simulink model "Robot4_SDT"  (R2025b)
settings: Solver=VariableStepAuto  StartTime=0.0  StopTime=10.0  RelTol=1e-3
values from neighbouring files (symbols this model uses):
  C_tile_force = 2*5*sqrt(K_tile_force*2.598*0.2*100)    [Satellite_Data.m]    (also in main.m)
  C_tile_torque = 2*1*sqrt(K_tile_torque*0.541266*100)*0.7    [Satellite_Data.m]    (also in main.m)
  CoM_variation_x = ureal('CoMx',0,"PlusMinus",[-10e-3 10e-3])    [Satellite_Data.m]
  CoM_variation_y = ureal('CoMy',0,"PlusMinus",[-10e-3 10e-3])    [Satellite_Data.m]
  CoM_variation_z = ureal('CoMz',0,"PlusMinus",[-20e-3 20e-3])    [Satellite_Data.m]
  Container_x = 1.5    [Satellite_Data.m]
  Container_z = sqrt(3)+0.5    [Satellite_Data.m]
  J_B_B = [J_B_Bxx J_B_Bxy J_B_Bxz;         J_B_Bxy J_B_Byy J_B_Byz;         J_B_Bxz J_B_Byz J_B_Bzz]    [Satellite_Data.m]
  J_C_C = [J_C_Cxx J_C_Cxy J_C_Cxz;         J_C_Cxy J_C_Cyy J_C_Cyz;         J_C_Cxz J_C_Cyz J_C_Czz]    [Satellite_Data.m]
  J_P_P = [J_P_Pxx J_P_Pxy J_P_Pxz;         J_P_Pxy J_P_Pyy J_P_Pyz;         J_P_Pxz J_P_Pyz J_P_Pzz]    [Satellite_Data.m]
  J_T_T = [J_T_Txx J_T_Txy J_T_Txz;          J_T_Txy J_T_Tyy J_T_Tyz;          J_T_Txz J_T_Tyz J_T_Tzz]    [Satellite_Data.m]
  K_tile_force = 2000/0.015    (= 133333.333333)    [Satellite_Data.m]    (also in main.m)
  K_tile_torque = 250/deg2rad(10)    [Satellite_Data.m]    (also in main.m)
  m_B = ureal('m_B',1000,'percent',10)    [Satellite_Data.m]
  m_C = ureal('m_C',500,'percent',10)    [Satellite_Data.m]
  m_P = ureal('m_P',50,'percent',2)    [Satellite_Data.m]
  m_T = ureal('m_T', m_nominal, 'percent', 2)    [Satellite_Data.m]
  robot = struct()    [Robotic_Arm_traj.m]    (also in Robotic_Arm_traj_no_energy.m; Satellite_Data.m; redundant_7dof_feasible_trajectory.m)
  Tile_z = 0.05    [Satellite_Data.m]
  unc_freq_boom = 10    [Satellite_Data.m]
undefined symbols (not defined in the file or in its folder): boom, InvDyn, InvDynAug, KIN, ureal, uss
libraries: SDTlibV1 x73, RCTblocks x39
(part 4 of 5)

== system Robot4_SDT/Tiles/Tile6/Variant Subsystem/Depose ==
  m_A : Inport
  m_C : Inport  Port=2
  m_T1 : Inport  Port=3
  m_T2 : Inport  Port=4
  m_EE : Inport  Port=5
  Constant : Constant
  Demux1 : Demux  Outputs=3
  Demux2 : Demux  Outputs=2
  Demux3 : Demux  Outputs=3
  Demux4 : Demux  Outputs=2
  Force : Subsystem
  Gain1 : Gain  Gain=-1
  Ground2 : Ground
  Integrator : Integrator
  Integrator1 : Integrator
  Mux : Mux
  Product : Product
  Product1 : Product
  Sum : Sum  Inputs=+-
  Sum1 : Sum  Inputs=|+-
  Terminator{,1..4} (5 alike) : Terminator
  Torque : Subsystem
  Zero : Constant  Value=zeros(6,1)  OutDataTypeStr=Inherit: Inherit via back propagation
  Zero1 : Constant  Value=zeros(6,1)  OutDataTypeStr=Inherit: Inherit via back propagation
  Zero2 : Constant  Value=zeros(6,1)  OutDataTypeStr=Inherit: Inherit via back propagation
  massless connection body : Subsystem  mask(Massless multi_port [6+18(n-1)]x[6(n-1)+18]){n=2, numinv=1, OP1=[0;0;0], OP2=[1.5 +sqrt(3)/2 0], OP3=[ureal('P3_y',1,'percent',10);0;0], OP4=[0;0;0], OP5=[0;0;0], OP6=[0;0;0], OP7=[0;0;0]}
      mask prompts: n "Number of ports"; numinv "Port (point) Pj: j="; OP1 "OP1 (3x1 vector, m)"; OP2 "OP2 (3x1 vector, m)"; OP3 "OP3 (3x1 vector, m)"; OP4 "OP4 (3x1 vector, m)"; OP5 "OP5 (3x1 vector,m)"; OP6 "OP6 (3x1 vector,m)"; OP7 "OP7 (3x1 vector,m)"
      mask help:
      | Massless body to transport wrenches and acceleration twists:
      | [6+18(n-1)]x[6(n-1)+18] gain from:
      |  * the motion vector at one point Pj; i.e. the parent port,
      |  * the wrenches applied to this massless body at the n-1 points Pi (i=1,..n, except j); i.e. the child ports
      | to:
      |  * the wrench applied at point Pj by this massless body,
      |  * the motion vectors at the other n-1  points Pi (i=1,..n, except j).
      |
      | 0: the reference point
      | Pi (i=1:n): the n given connection points or ports (1<n<8).
      |
      | All parameters are expressed in the body frame.
      | Each parameter can be an uncertain parameter declared with "ureal"
      mask init:
      | MasslessConnectionBodyAug
      mask Help: web('DocMassLessBody.html','-browser','-browser')
      mask TypeOptions n: 2 | 3 | 4 | 5 | 6 | 7
      mask TypeOptions numinv: 1 | 2 | 3 | 4 | 5 | 6 | 7
      mask DialogControl ParameterGroupVar Prompt: Main parameters
      mask DialogControl port1 Prompt: Port #1
      mask DialogControl port2 Prompt: #2
      mask DialogControl port3 Prompt: #3
      mask DialogControl port4 Prompt: #4
      mask DialogControl port5 Prompt: #5
      mask DialogControl port6 Prompt: #6
      mask DialogControl port7 Prompt: #7
      mask Display:
      | disp('Massless\n connection body\n [6+18(n-1)]x[6(n-1)+18]')
      | for ii=1:n+1
      |     if numinv==ii,
      |         port_label('output',ii,['Wbody/.,P',num2str(ii)])
      |         port_label('input', ii,['m_P',num2str(ii)])
      |     else
      |         port_label('input', ii,['W./body,P',num2str(ii)])
      |         port_label('output',ii,['m_P',num2str(ii)])
      |     end
      | end
  W_A : Outport
  W_C : Outport  Port=2
  W_T1 : Outport  Port=3
  W_T2 : Outport  Port=4
  W_EE : Outport  Port=5
  wires:
  Force/1(Mating) -> Product1/2
  Constant/1 -> Product/2, Product1/1
  Demux3/3 -> [Fz]
  Demux3/1 -> [Fx]
  Demux3/2 -> [Fy]
  Product/1 -> [T]
  Torque/1(Mating) -> Product/1
  Product1/1 -> Demux3/1
  Demux4/2 -> Torque/1(EA)
  Demux4/1 -> Force/1(pos)
  [T] -> Mux/4
  Demux1/3 -> Terminator3/1
  Integrator1/1 -> Demux4/1
  [Fy] -> Mux/2
  Demux1/1 -> Integrator/1
  Gain1/1 -> Demux1/1
  massless connection body/2(out2) -> Sum/1
  [Fz] -> Mux/3
  Sum1/1 -> massless connection body/2(in2)
  Mux/1 -> Sum1/2, W_T1/1
  Demux1/2 -> Terminator2/1
  Demux2/2 -> Torque/2(Omega)
  [Fx] -> Mux/1
  Integrator/1 -> Demux2/1, Integrator1/1
  Ground2/1 -> Sum1/1
  Demux2/1 -> Force/2(vel)
  Sum/1 -> Gain1/1
  m_T1/1 -> Sum/2
  m_A/1 -> massless connection body/1(in1)
  massless connection body/1(out1) -> W_A/1
  m_T2/1 -> Terminator1/1
  m_EE/1 -> Terminator/1
  m_C/1 -> Terminator4/1
  Zero/1 -> W_EE/1
  Zero1/1 -> W_T2/1
  Zero2/1 -> W_C/1

== system Robot4_SDT/Tiles/Tile6/Variant Subsystem/Grab ==
  m_EE : Inport
  m_C : Inport  Port=2
  m_T2 : Inport  Port=3
  m_A : Inport  Port=4
  m_T1 : Inport  Port=5
  Demux1 : Demux  Outputs=3
  Demux2 : Demux  Outputs=2
  Demux3 : Demux  Outputs=3
  Demux4 : Demux  Outputs=2
  Force : Subsystem
  Gain1 : Gain  Gain=-1
  Ground2 : Ground
  Integrator : Integrator
  Integrator1 : Integrator
  Mux : Mux
  Sum : Sum  Inputs=+-
  Sum1 : Sum  Inputs=|+-
  Terminator{,1..4} (5 alike) : Terminator
  Torque : Subsystem
  Zero : Constant  Value=zeros(6,1)  OutDataTypeStr=Inherit: Inherit via back propagation
  Zero1 : Constant  Value=zeros(6,1)  OutDataTypeStr=Inherit: Inherit via back propagation
  Zero2 : Constant  Value=zeros(6,1)  OutDataTypeStr=Inherit: Inherit via back propagation
  massless connection body : Subsystem  mask(Massless multi_port [6+18(n-1)]x[6(n-1)+18]){n=2, numinv=1, OP1=[0;0;0], OP2=[0;0;0], OP3=[ureal('P3_y',1,'percent',10);0;0], OP4=[0;0;0], OP5=[0;0;0], OP6=[0;0;0], OP7=[0;0;0]}
      mask prompts: n "Number of ports"; numinv "Port (point) Pj: j="; OP1 "OP1 (3x1 vector, m)"; OP2 "OP2 (3x1 vector, m)"; OP3 "OP3 (3x1 vector, m)"; OP4 "OP4 (3x1 vector, m)"; OP5 "OP5 (3x1 vector,m)"; OP6 "OP6 (3x1 vector,m)"; OP7 "OP7 (3x1 vector,m)"
      mask help:
      | Massless body to transport wrenches and acceleration twists:
      | [6+18(n-1)]x[6(n-1)+18] gain from:
      |  * the motion vector at one point Pj; i.e. the parent port,
      |  * the wrenches applied to this massless body at the n-1 points Pi (i=1,..n, except j); i.e. the child ports
      | to:
      |  * the wrench applied at point Pj by this massless body,
      |  * the motion vectors at the other n-1  points Pi (i=1,..n, except j).
      |
      | 0: the reference point
      | Pi (i=1:n): the n given connection points or ports (1<n<8).
      |
      | All parameters are expressed in the body frame.
      | Each parameter can be an uncertain parameter declared with "ureal"
      mask init:
      | MasslessConnectionBodyAug
      mask Help: web('DocMassLessBody.html','-browser','-browser')
      mask TypeOptions n: 2 | 3 | 4 | 5 | 6 | 7
      mask TypeOptions numinv: 1 | 2 | 3 | 4 | 5 | 6 | 7
      mask DialogControl ParameterGroupVar Prompt: Main parameters
      mask DialogControl port1 Prompt: Port #1
      mask DialogControl port2 Prompt: #2
      mask DialogControl port3 Prompt: #3
      mask DialogControl port4 Prompt: #4
      mask DialogControl port5 Prompt: #5
      mask DialogControl port6 Prompt: #6
      mask DialogControl port7 Prompt: #7
      mask Display:
      | disp('Massless\n connection body\n [6+18(n-1)]x[6(n-1)+18]')
      | for ii=1:n+1
      |     if numinv==ii,
      |         port_label('output',ii,['Wbody/.,P',num2str(ii)])
      |         port_label('input', ii,['m_P',num2str(ii)])
      |     else
      |         port_label('input', ii,['W./body,P',num2str(ii)])
      |         port_label('output',ii,['m_P',num2str(ii)])
      |     end
      | end
  W_EE : Outport
  W_C : Outport  Port=2
  W_T2 : Outport  Port=3
  W_A : Outport  Port=4
  W_T1 : Outport  Port=5
  wires:
  Torque/1(Mating) -> [T]
  massless connection body/1(out1) -> W_EE/1
  m_EE/1 -> massless connection body/1(in1)
  m_T2/1 -> Sum/2
  Sum/1 -> Gain1/1
  Demux2/1 -> Force/2(vel)
  Ground2/1 -> Sum1/1
  Integrator/1 -> Integrator1/1, Demux2/1
  [Fx] -> Mux/1
  Demux2/2 -> Torque/2(Omega)
  Demux1/2 -> Terminator2/1
  Mux/1 -> W_T2/1, Sum1/2
  Sum1/1 -> massless connection body/2(in2)
  [Fz] -> Mux/3
  massless connection body/2(out2) -> Sum/1
  Gain1/1 -> Demux1/1
  Demux1/1 -> Integrator/1
  [Fy] -> Mux/2
  Integrator1/1 -> Demux4/1
  Demux1/3 -> Terminator3/1
  [T] -> Mux/4
  Demux4/1 -> Force/1(pos)
  Demux4/2 -> Torque/1(EA)
  Force/1(Mating) -> Demux3/1
  Demux3/2 -> [Fy]
  Demux3/1 -> [Fx]
  Demux3/3 -> [Fz]
  m_A/1 -> Terminator1/1
  m_C/1 -> Terminator/1
  m_T1/1 -> Terminator4/1
  Zero/1 -> W_C/1
  Zero1/1 -> W_A/1
  Zero2/1 -> W_T1/1

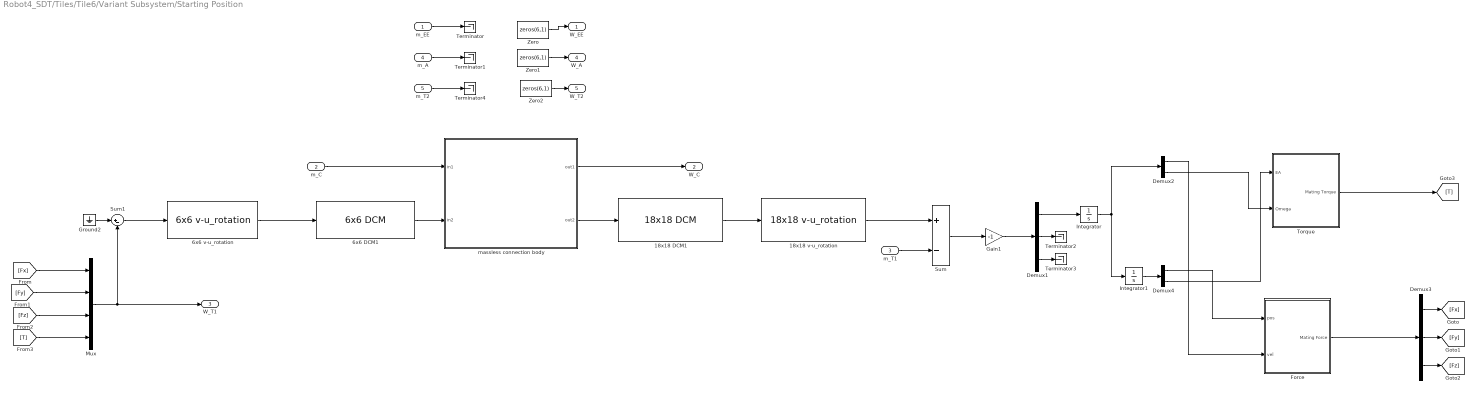
== system Robot4_SDT/Tiles/Tile6/Variant Subsystem/Starting Position ==
  m_EE : Inport
  m_C : Inport  Port=2
  m_T1 : Inport  Port=3
  m_A : Inport  Port=4
  m_T2 : Inport  Port=5
  18x18 DCM1 : SDTlibV1/3//6//18 DCM/18x18 DCM  rot=[0 0 1;0 1 0;-1 0 0]  transp=on
      settings: SourceProductName=SDTlib
  18x18 v-u_rotation : SDTlibV1/3//6//18 DCM/18x18 v-u_rotation  ra=[0;0;1]  theta=pi/2  transp=on
      settings: SourceProductName=SDTlib
  6x6 DCM1 : SDTlibV1/3//6//18 DCM/6x6 DCM  rot=[0 0 1;0 1 0;-1 0 0]  transp=off
      settings: SourceProductName=SDTlib
  6x6 v-u_rotation : SDTlibV1/3//6//18 DCM/6x6 v-u_rotation  ra=[0;0;1]  theta=pi/2  transp=off
      settings: SourceProductName=SDTlib
  Demux1 : Demux  Outputs=3
  Demux2 : Demux  Outputs=2
  Demux3 : Demux  Outputs=3
  Demux4 : Demux  Outputs=2
  Force : Subsystem
  Gain1 : Gain  Gain=-1
  Ground2 : Ground
  Integrator : Integrator
  Integrator1 : Integrator
  Mux : Mux
  Sum : Sum  Inputs=+-
  Sum1 : Sum  Inputs=|+-
  Terminator{,1..4} (5 alike) : Terminator
  Torque : Subsystem
  Zero : Constant  Value=zeros(6,1)  OutDataTypeStr=Inherit: Inherit via back propagation
  Zero1 : Constant  Value=zeros(6,1)  OutDataTypeStr=Inherit: Inherit via back propagation
  Zero2 : Constant  Value=zeros(6,1)  OutDataTypeStr=Inherit: Inherit via back propagation
  massless connection body : Subsystem  mask(Massless multi_port [6+18(n-1)]x[6(n-1)+18]){n=2, numinv=1, OP1=[0;0;0], OP2=[-1.2;0;0], OP3=[ureal('P3_y',1,'percent',10);0;0], OP4=[0;0;0], OP5=[0;0;0], OP6=[0;0;0], OP7=[0;0;0]}
      mask prompts: n "Number of ports"; numinv "Port (point) Pj: j="; OP1 "OP1 (3x1 vector, m)"; OP2 "OP2 (3x1 vector, m)"; OP3 "OP3 (3x1 vector, m)"; OP4 "OP4 (3x1 vector, m)"; OP5 "OP5 (3x1 vector,m)"; OP6 "OP6 (3x1 vector,m)"; OP7 "OP7 (3x1 vector,m)"
      mask help:
      | Massless body to transport wrenches and acceleration twists:
      | [6+18(n-1)]x[6(n-1)+18] gain from:
      |  * the motion vector at one point Pj; i.e. the parent port,
      |  * the wrenches applied to this massless body at the n-1 points Pi (i=1,..n, except j); i.e. the child ports
      | to:
      |  * the wrench applied at point Pj by this massless body,
      |  * the motion vectors at the other n-1  points Pi (i=1,..n, except j).
      |
      | 0: the reference point
      | Pi (i=1:n): the n given connection points or ports (1<n<8).
      |
      | All parameters are expressed in the body frame.
      | Each parameter can be an uncertain parameter declared with "ureal"
      mask init:
      | MasslessConnectionBodyAug
      mask Help: web('DocMassLessBody.html','-browser','-browser')
      mask TypeOptions n: 2 | 3 | 4 | 5 | 6 | 7
      mask TypeOptions numinv: 1 | 2 | 3 | 4 | 5 | 6 | 7
      mask DialogControl ParameterGroupVar Prompt: Main parameters
      mask DialogControl port1 Prompt: Port #1
      mask DialogControl port2 Prompt: #2
      mask DialogControl port3 Prompt: #3
      mask DialogControl port4 Prompt: #4
      mask DialogControl port5 Prompt: #5
      mask DialogControl port6 Prompt: #6
      mask DialogControl port7 Prompt: #7
      mask Display:
      | disp('Massless\n connection body\n [6+18(n-1)]x[6(n-1)+18]')
      | for ii=1:n+1
      |     if numinv==ii,
      |         port_label('output',ii,['Wbody/.,P',num2str(ii)])
      |         port_label('input', ii,['m_P',num2str(ii)])
      |     else
      |         port_label('input', ii,['W./body,P',num2str(ii)])
      |         port_label('output',ii,['m_P',num2str(ii)])
      |     end
      | end
  W_EE : Outport
  W_C : Outport  Port=2
  W_T1 : Outport  Port=3
  W_A : Outport  Port=4
  W_T2 : Outport  Port=5
  wires:
  Demux3/3 -> [Fz]
  Demux3/1 -> [Fx]
  Demux3/2 -> [Fy]
  Torque/1(Mating Torque) -> [T]
  Force/1(Mating Force) -> Demux3/1
  massless connection body/1(out1) -> W_C/1
  m_C/1 -> massless connection body/1(in1)
  m_T1/1 -> Sum/2
  Sum/1 -> Gain1/1
  Demux2/1 -> Force/2(vel)
  Ground2/1 -> Sum1/1
  Integrator/1 -> Integrator1/1, Demux2/1
  [Fx] -> Mux/1
  Demux2/2 -> Torque/2(Omega)
  Demux1/2 -> Terminator2/1
  Mux/1 -> Sum1/2, W_T1/1
  6x6 DCM1/1 -> massless connection body/2(in2)
  18x18 DCM1/1 -> 18x18 v-u_rotation/1
  Sum1/1 -> 6x6 v-u_rotation/1
  [Fz] -> Mux/3
  18x18 v-u_rotation/1 -> Sum/1
  Gain1/1 -> Demux1/1
  Demux1/1 -> Integrator/1
  6x6 v-u_rotation/1 -> 6x6 DCM1/1
  [Fy] -> Mux/2
  massless connection body/2(out2) -> 18x18 DCM1/1
  Integrator1/1 -> Demux4/1
  Demux1/3 -> Terminator3/1
  [T] -> Mux/4
  Demux4/1 -> Force/1(pos)
  Demux4/2 -> Torque/1(EA)
  m_A/1 -> Terminator1/1
  m_EE/1 -> Terminator/1
  m_T2/1 -> Terminator4/1
  Zero/1 -> W_EE/1
  Zero1/1 -> W_A/1
  Zero2/1 -> W_T2/1

== system Robot4_SDT/Tiles/Tile7/Variant Subsystem/Depose ==
  m_A : Inport
  m_C : Inport  Port=2
  m_T1 : Inport  Port=3
  m_T2 : Inport  Port=4
  m_EE : Inport  Port=5
  Constant : Constant
  Demux1 : Demux  Outputs=3
  Demux2 : Demux  Outputs=2
  Demux3 : Demux  Outputs=3
  Demux4 : Demux  Outputs=2
  Force : Subsystem
  Gain1 : Gain  Gain=-1
  Ground2 : Ground
  Integrator : Integrator
  Integrator1 : Integrator
  Mux : Mux
  Product : Product
  Product1 : Product
  Sum : Sum  Inputs=+-
  Sum1 : Sum  Inputs=|+-
  Terminator{,1..4} (5 alike) : Terminator
  Torque : Subsystem
  Zero : Constant  Value=zeros(6,1)  OutDataTypeStr=Inherit: Inherit via back propagation
  Zero1 : Constant  Value=zeros(6,1)  OutDataTypeStr=Inherit: Inherit via back propagation
  Zero2 : Constant  Value=zeros(6,1)  OutDataTypeStr=Inherit: Inherit via back propagation
  massless connection body : Subsystem  mask(Massless multi_port [6+18(n-1)]x[6(n-1)+18]){n=2, numinv=1, OP1=[0;0;0], OP2=[1.5 -sqrt(3)/2 0], OP3=[ureal('P3_y',1,'percent',10);0;0], OP4=[0;0;0], OP5=[0;0;0], OP6=[0;0;0], OP7=[0;0;0]}
      mask prompts: n "Number of ports"; numinv "Port (point) Pj: j="; OP1 "OP1 (3x1 vector, m)"; OP2 "OP2 (3x1 vector, m)"; OP3 "OP3 (3x1 vector, m)"; OP4 "OP4 (3x1 vector, m)"; OP5 "OP5 (3x1 vector,m)"; OP6 "OP6 (3x1 vector,m)"; OP7 "OP7 (3x1 vector,m)"
      mask help:
      | Massless body to transport wrenches and acceleration twists:
      | [6+18(n-1)]x[6(n-1)+18] gain from:
      |  * the motion vector at one point Pj; i.e. the parent port,
      |  * the wrenches applied to this massless body at the n-1 points Pi (i=1,..n, except j); i.e. the child ports
      | to:
      |  * the wrench applied at point Pj by this massless body,
      |  * the motion vectors at the other n-1  points Pi (i=1,..n, except j).
      |
      | 0: the reference point
      | Pi (i=1:n): the n given connection points or ports (1<n<8).
      |
      | All parameters are expressed in the body frame.
      | Each parameter can be an uncertain parameter declared with "ureal"
      mask init:
      | MasslessConnectionBodyAug
      mask Help: web('DocMassLessBody.html','-browser','-browser')
      mask TypeOptions n: 2 | 3 | 4 | 5 | 6 | 7
      mask TypeOptions numinv: 1 | 2 | 3 | 4 | 5 | 6 | 7
      mask DialogControl ParameterGroupVar Prompt: Main parameters
      mask DialogControl port1 Prompt: Port #1
      mask DialogControl port2 Prompt: #2
      mask DialogControl port3 Prompt: #3
      mask DialogControl port4 Prompt: #4
      mask DialogControl port5 Prompt: #5
      mask DialogControl port6 Prompt: #6
      mask DialogControl port7 Prompt: #7
      mask Display:
      | disp('Massless\n connection body\n [6+18(n-1)]x[6(n-1)+18]')
      | for ii=1:n+1
      |     if numinv==ii,
      |         port_label('output',ii,['Wbody/.,P',num2str(ii)])
      |         port_label('input', ii,['m_P',num2str(ii)])
      |     else
      |         port_label('input', ii,['W./body,P',num2str(ii)])
      |         port_label('output',ii,['m_P',num2str(ii)])
      |     end
      | end
  W_A : Outport
  W_C : Outport  Port=2
  W_T1 : Outport  Port=3
  W_T2 : Outport  Port=4
  W_EE : Outport  Port=5
  wires:
  Zero2/1 -> W_C/1
  Zero1/1 -> W_T2/1
  Zero/1 -> W_EE/1
  m_C/1 -> Terminator4/1
  m_EE/1 -> Terminator/1
  m_T2/1 -> Terminator1/1
  massless connection body/1(out1) -> W_A/1
  m_A/1 -> massless connection body/1(in1)
  m_T1/1 -> Sum/2
  Sum/1 -> Gain1/1
  Demux2/1 -> Force/2(vel)
  Ground2/1 -> Sum1/1
  Integrator/1 -> Integrator1/1, Demux2/1
  [Fx] -> Mux/1
  Demux2/2 -> Torque/2(Omega)
  Demux1/2 -> Terminator2/1
  Mux/1 -> W_T1/1, Sum1/2
  Sum1/1 -> massless connection body/2(in2)
  [Fz] -> Mux/3
  massless connection body/2(out2) -> Sum/1
  Gain1/1 -> Demux1/1
  Demux1/1 -> Integrator/1
  [Fy] -> Mux/2
  Integrator1/1 -> Demux4/1
  Demux1/3 -> Terminator3/1
  [T] -> Mux/4
  Demux4/1 -> Force/1(pos)
  Demux4/2 -> Torque/1(EA)
  Product1/1 -> Demux3/1
  Torque/1(Mating) -> Product/1
  Product/1 -> [T]
  Demux3/2 -> [Fy]
  Demux3/1 -> [Fx]
  Demux3/3 -> [Fz]
  Constant/1 -> Product1/1, Product/2
  Force/1(Mating) -> Product1/2

== system Robot4_SDT/Tiles/Tile7/Variant Subsystem/Grab ==
  m_EE : Inport
  m_C : Inport  Port=2
  m_T2 : Inport  Port=3
  m_A : Inport  Port=4
  m_T1 : Inport  Port=5
  Demux1 : Demux  Outputs=3
  Demux2 : Demux  Outputs=2
  Demux3 : Demux  Outputs=3
  Demux4 : Demux  Outputs=2
  Force : Subsystem
  Gain1 : Gain  Gain=-1
  Ground2 : Ground
  Integrator : Integrator
  Integrator1 : Integrator
  Mux : Mux
  Sum : Sum  Inputs=+-
  Sum1 : Sum  Inputs=|+-
  Terminator{,1..4} (5 alike) : Terminator
  Torque : Subsystem
  Zero : Constant  Value=zeros(6,1)  OutDataTypeStr=Inherit: Inherit via back propagation
  Zero1 : Constant  Value=zeros(6,1)  OutDataTypeStr=Inherit: Inherit via back propagation
  Zero2 : Constant  Value=zeros(6,1)  OutDataTypeStr=Inherit: Inherit via back propagation
  massless connection body : Subsystem  mask(Massless multi_port [6+18(n-1)]x[6(n-1)+18]){n=2, numinv=1, OP1=[0;0;0], OP2=[0;0;0], OP3=[ureal('P3_y',1,'percent',10);0;0], OP4=[0;0;0], OP5=[0;0;0], OP6=[0;0;0], OP7=[0;0;0]}
      mask prompts: n "Number of ports"; numinv "Port (point) Pj: j="; OP1 "OP1 (3x1 vector, m)"; OP2 "OP2 (3x1 vector, m)"; OP3 "OP3 (3x1 vector, m)"; OP4 "OP4 (3x1 vector, m)"; OP5 "OP5 (3x1 vector,m)"; OP6 "OP6 (3x1 vector,m)"; OP7 "OP7 (3x1 vector,m)"
      mask help:
      | Massless body to transport wrenches and acceleration twists:
      | [6+18(n-1)]x[6(n-1)+18] gain from:
      |  * the motion vector at one point Pj; i.e. the parent port,
      |  * the wrenches applied to this massless body at the n-1 points Pi (i=1,..n, except j); i.e. the child ports
      | to:
      |  * the wrench applied at point Pj by this massless body,
      |  * the motion vectors at the other n-1  points Pi (i=1,..n, except j).
      |
      | 0: the reference point
      | Pi (i=1:n): the n given connection points or ports (1<n<8).
      |
      | All parameters are expressed in the body frame.
      | Each parameter can be an uncertain parameter declared with "ureal"
      mask init:
      | MasslessConnectionBodyAug
      mask Help: web('DocMassLessBody.html','-browser','-browser')
      mask TypeOptions n: 2 | 3 | 4 | 5 | 6 | 7
      mask TypeOptions numinv: 1 | 2 | 3 | 4 | 5 | 6 | 7
      mask DialogControl ParameterGroupVar Prompt: Main parameters
      mask DialogControl port1 Prompt: Port #1
      mask DialogControl port2 Prompt: #2
      mask DialogControl port3 Prompt: #3
      mask DialogControl port4 Prompt: #4
      mask DialogControl port5 Prompt: #5
      mask DialogControl port6 Prompt: #6
      mask DialogControl port7 Prompt: #7
      mask Display:
      | disp('Massless\n connection body\n [6+18(n-1)]x[6(n-1)+18]')
      | for ii=1:n+1
      |     if numinv==ii,
      |         port_label('output',ii,['Wbody/.,P',num2str(ii)])
      |         port_label('input', ii,['m_P',num2str(ii)])
      |     else
      |         port_label('input', ii,['W./body,P',num2str(ii)])
      |         port_label('output',ii,['m_P',num2str(ii)])
      |     end
      | end
  W_EE : Outport
  W_C : Outport  Port=2
  W_T2 : Outport  Port=3
  W_A : Outport  Port=4
  W_T1 : Outport  Port=5
  wires:
  Zero2/1 -> W_T1/1
  Zero1/1 -> W_A/1
  Zero/1 -> W_C/1
  m_T1/1 -> Terminator4/1
  m_C/1 -> Terminator/1
  m_A/1 -> Terminator1/1
  Demux3/3 -> [Fz]
  Demux3/1 -> [Fx]
  Demux3/2 -> [Fy]
  Force/1(Mating) -> Demux3/1
  Demux4/2 -> Torque/1(EA)
  Demux4/1 -> Force/1(pos)
  [T] -> Mux/4
  Demux1/3 -> Terminator3/1
  Integrator1/1 -> Demux4/1
  [Fy] -> Mux/2
  Demux1/1 -> Integrator/1
  Gain1/1 -> Demux1/1
  massless connection body/2(out2) -> Sum/1
  [Fz] -> Mux/3
  Sum1/1 -> massless connection body/2(in2)
  Mux/1 -> Sum1/2, W_T2/1
  Demux1/2 -> Terminator2/1
  Demux2/2 -> Torque/2(Omega)
  [Fx] -> Mux/1
  Integrator/1 -> Demux2/1, Integrator1/1
  Ground2/1 -> Sum1/1
  Demux2/1 -> Force/2(vel)
  Sum/1 -> Gain1/1
  m_T2/1 -> Sum/2
  m_EE/1 -> massless connection body/1(in1)
  massless connection body/1(out1) -> W_EE/1
  Torque/1(Mating) -> [T]

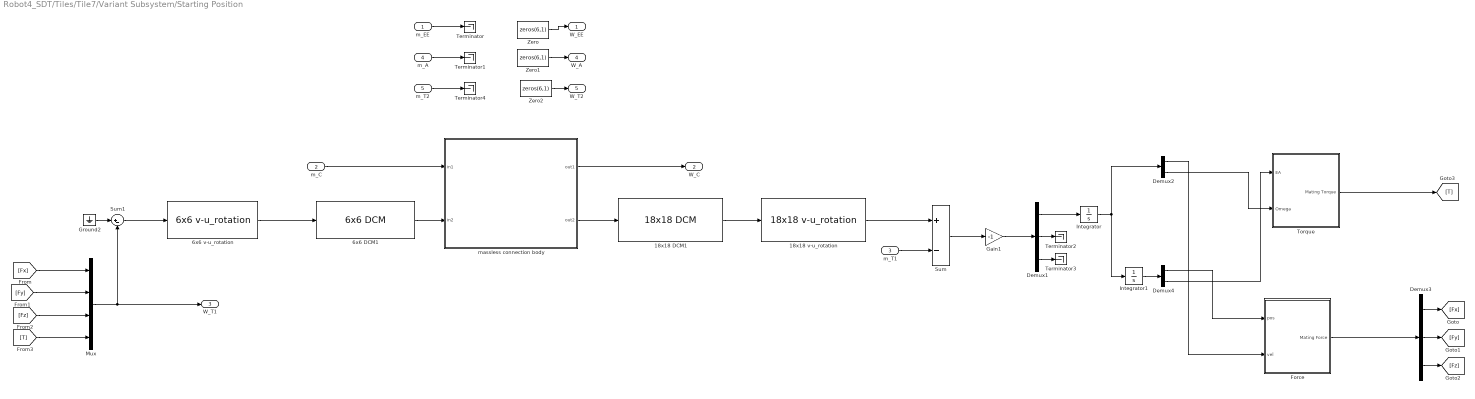
== system Robot4_SDT/Tiles/Tile7/Variant Subsystem/Starting Position ==
  m_EE : Inport
  m_C : Inport  Port=2
  m_T1 : Inport  Port=3
  m_A : Inport  Port=4
  m_T2 : Inport  Port=5
  18x18 DCM1 : SDTlibV1/3//6//18 DCM/18x18 DCM  rot=[0 0 1;0 1 0;-1 0 0]  transp=on
      settings: SourceProductName=SDTlib
  18x18 v-u_rotation : SDTlibV1/3//6//18 DCM/18x18 v-u_rotation  ra=[0;0;1]  theta=pi/2  transp=on
      settings: SourceProductName=SDTlib
  6x6 DCM1 : SDTlibV1/3//6//18 DCM/6x6 DCM  rot=[0 0 1;0 1 0;-1 0 0]  transp=off
      settings: SourceProductName=SDTlib
  6x6 v-u_rotation : SDTlibV1/3//6//18 DCM/6x6 v-u_rotation  ra=[0;0;1]  theta=pi/2  transp=off
      settings: SourceProductName=SDTlib
  Demux1 : Demux  Outputs=3
  Demux2 : Demux  Outputs=2
  Demux3 : Demux  Outputs=3
  Demux4 : Demux  Outputs=2
  Force : Subsystem
  Gain1 : Gain  Gain=-1
  Ground2 : Ground
  Integrator : Integrator
  Integrator1 : Integrator
  Mux : Mux
  Sum : Sum  Inputs=+-
  Sum1 : Sum  Inputs=|+-
  Terminator{,1..4} (5 alike) : Terminator
  Torque : Subsystem
  Zero : Constant  Value=zeros(6,1)  OutDataTypeStr=Inherit: Inherit via back propagation
  Zero1 : Constant  Value=zeros(6,1)  OutDataTypeStr=Inherit: Inherit via back propagation
  Zero2 : Constant  Value=zeros(6,1)  OutDataTypeStr=Inherit: Inherit via back propagation
  massless connection body : Subsystem  mask(Massless multi_port [6+18(n-1)]x[6(n-1)+18]){n=2, numinv=1, OP1=[0;0;0], OP2=[-1.4;0;0], OP3=[ureal('P3_y',1,'percent',10);0;0], OP4=[0;0;0], OP5=[0;0;0], OP6=[0;0;0], OP7=[0;0;0]}
      mask prompts: n "Number of ports"; numinv "Port (point) Pj: j="; OP1 "OP1 (3x1 vector, m)"; OP2 "OP2 (3x1 vector, m)"; OP3 "OP3 (3x1 vector, m)"; OP4 "OP4 (3x1 vector, m)"; OP5 "OP5 (3x1 vector,m)"; OP6 "OP6 (3x1 vector,m)"; OP7 "OP7 (3x1 vector,m)"
      mask help:
      | Massless body to transport wrenches and acceleration twists:
      | [6+18(n-1)]x[6(n-1)+18] gain from:
      |  * the motion vector at one point Pj; i.e. the parent port,
      |  * the wrenches applied to this massless body at the n-1 points Pi (i=1,..n, except j); i.e. the child ports
      | to:
      |  * the wrench applied at point Pj by this massless body,
      |  * the motion vectors at the other n-1  points Pi (i=1,..n, except j).
      |
      | 0: the reference point
      | Pi (i=1:n): the n given connection points or ports (1<n<8).
      |
      | All parameters are expressed in the body frame.
      | Each parameter can be an uncertain parameter declared with "ureal"
      mask init:
      | MasslessConnectionBodyAug
      mask Help: web('DocMassLessBody.html','-browser','-browser')
      mask TypeOptions n: 2 | 3 | 4 | 5 | 6 | 7
      mask TypeOptions numinv: 1 | 2 | 3 | 4 | 5 | 6 | 7
      mask DialogControl ParameterGroupVar Prompt: Main parameters
      mask DialogControl port1 Prompt: Port #1
      mask DialogControl port2 Prompt: #2
      mask DialogControl port3 Prompt: #3
      mask DialogControl port4 Prompt: #4
      mask DialogControl port5 Prompt: #5
      mask DialogControl port6 Prompt: #6
      mask DialogControl port7 Prompt: #7
      mask Display:
      | disp('Massless\n connection body\n [6+18(n-1)]x[6(n-1)+18]')
      | for ii=1:n+1
      |     if numinv==ii,
      |         port_label('output',ii,['Wbody/.,P',num2str(ii)])
      |         port_label('input', ii,['m_P',num2str(ii)])
      |     else
      |         port_label('input', ii,['W./body,P',num2str(ii)])
      |         port_label('output',ii,['m_P',num2str(ii)])
      |     end
      | end
  W_EE : Outport
  W_C : Outport  Port=2
  W_T1 : Outport  Port=3
  W_A : Outport  Port=4
  W_T2 : Outport  Port=5
  wires:
  Zero2/1 -> W_T2/1
  Zero1/1 -> W_A/1
  Zero/1 -> W_EE/1
  m_T2/1 -> Terminator4/1
  m_EE/1 -> Terminator/1
  m_A/1 -> Terminator1/1
  Demux4/2 -> Torque/1(EA)
  Demux4/1 -> Force/1(pos)
  [T] -> Mux/4
  Demux1/3 -> Terminator3/1
  Integrator1/1 -> Demux4/1
  massless connection body/2(out2) -> 18x18 DCM1/1
  [Fy] -> Mux/2
  6x6 v-u_rotation/1 -> 6x6 DCM1/1
  Demux1/1 -> Integrator/1
  Gain1/1 -> Demux1/1
  18x18 v-u_rotation/1 -> Sum/1
  [Fz] -> Mux/3
  Sum1/1 -> 6x6 v-u_rotation/1
  18x18 DCM1/1 -> 18x18 v-u_rotation/1
  6x6 DCM1/1 -> massless connection body/2(in2)
  Mux/1 -> W_T1/1, Sum1/2
  Demux1/2 -> Terminator2/1
  Demux2/2 -> Torque/2(Omega)
  [Fx] -> Mux/1
  Integrator/1 -> Demux2/1, Integrator1/1
  Ground2/1 -> Sum1/1
  Demux2/1 -> Force/2(vel)
  Sum/1 -> Gain1/1
  m_T1/1 -> Sum/2
  m_C/1 -> massless connection body/1(in1)
  massless connection body/1(out1) -> W_C/1
  Force/1(Mating Force) -> Demux3/1
  Torque/1(Mating Torque) -> [T]
  Demux3/2 -> [Fy]
  Demux3/1 -> [Fx]
  Demux3/3 -> [Fz]

== system Robot4_SDT/Tiles/Tile1/Variant Subsystem/Depose/Force ==
  pos : Inport
  vel : Inport  Port=2
  Constant : Constant  Value=K_tile_force
  Constant1 : Constant  Value=C_tile_force
  Product : Product
  Product1 : Product
  Sum : Sum  Inputs=--
  Mating : Outport
  wires:
  vel/1 -> Product1/1
  pos/1 -> Product/2
  Sum/1 -> Mating/1
  Product1/1 -> Sum/2
  Product/1 -> Sum/1
  Constant1/1 -> Product1/2
  Constant/1 -> Product/1

== system Robot4_SDT/Tiles/Tile1/Variant Subsystem/Depose/Torque ==
  EA : Inport
  Omega : Inport  Port=2
  Constant : Constant  Value=K_tile_torque
  Constant1 : Constant  Value=C_tile_torque
  Product : Product
  Product1 : Product
  Sum : Sum  Inputs=--
  Mating : Outport
  wires:
  Omega/1 -> Product1/1
  EA/1 -> Product/2
  Sum/1 -> Mating/1
  Product1/1 -> Sum/2
  Product/1 -> Sum/1
  Constant1/1 -> Product1/2
  Constant/1 -> Product/1

== system Robot4_SDT/Tiles/Tile1/Variant Subsystem/Depose/massless connection body ==
  in1 : Inport  PortDimensions=18
  in2 : Inport  Port=2  PortDimensions=6
  Demux : Demux  Outputs=[ 6 18]
  Gain : RCTblocks/Uncertain State Space  Tag=USS  USystem=uss(KIN)  UValue=[]  X0=[]  uX0=[]
  Mux : Mux  Inputs=[ 18 6]
  out1 : Outport
  out2 : Outport  Port=2
  wires:
  Demux/2 -> out2/1
  in2/1 -> Mux/2
  Demux/1 -> out1/1
  in1/1 -> Mux/1
  Gain/1 -> Demux/1
  Mux/1 -> Gain/1

== system Robot4_SDT/Tiles/Tile1/Variant Subsystem/Grab/Force ==
  pos : Inport
  vel : Inport  Port=2
  Constant : Constant  Value=K_tile_force
  Constant1 : Constant  Value=C_tile_force
  Product : Product
  Product1 : Product
  Sum : Sum  Inputs=--
  Mating : Outport
  wires:
  Constant/1 -> Product/1
  Constant1/1 -> Product1/2
  Product/1 -> Sum/1
  Product1/1 -> Sum/2
  Sum/1 -> Mating/1
  pos/1 -> Product/2
  vel/1 -> Product1/1

== system Robot4_SDT/Tiles/Tile1/Variant Subsystem/Grab/Torque ==
  EA : Inport
  Omega : Inport  Port=2
  Constant : Constant  Value=K_tile_torque
  Constant1 : Constant  Value=C_tile_torque
  Product : Product
  Product1 : Product
  Sum : Sum  Inputs=--
  Mating : Outport
  wires:
  Constant/1 -> Product/1
  Constant1/1 -> Product1/2
  Product/1 -> Sum/1
  Product1/1 -> Sum/2
  Sum/1 -> Mating/1
  EA/1 -> Product/2
  Omega/1 -> Product1/1

== system Robot4_SDT/Tiles/Tile1/Variant Subsystem/Grab/massless connection body ==
  in1 : Inport  PortDimensions=18
  in2 : Inport  Port=2  PortDimensions=6
  Demux : Demux  Outputs=[ 6 18]
  Gain : RCTblocks/Uncertain State Space  Tag=USS  USystem=uss(KIN)  UValue=[]  X0=[]  uX0=[]
  Mux : Mux  Inputs=[ 18 6]
  out1 : Outport
  out2 : Outport  Port=2
  wires:
  Mux/1 -> Gain/1
  Gain/1 -> Demux/1
  in1/1 -> Mux/1
  Demux/1 -> out1/1
  in2/1 -> Mux/2
  Demux/2 -> out2/1

== system Robot4_SDT/Tiles/Tile1/Variant Subsystem/Starting Position/Force ==
  pos : Inport
  vel : Inport  Port=2
  Constant : Constant  Value=150000
  Constant1 : Constant  Value=8000
  Product : Product
  Product1 : Product
  Sum : Sum  Inputs=--
  Mating Force : Outport
  wires:
  Constant/1 -> Product/1
  Constant1/1 -> Product1/2
  Product/1 -> Sum/1
  Product1/1 -> Sum/2
  Sum/1 -> Mating Force/1
  pos/1 -> Product/2
  vel/1 -> Product1/1

== system Robot4_SDT/Tiles/Tile1/Variant Subsystem/Starting Position/Torque ==
  EA : Inport
  Omega : Inport  Port=2
  Constant : Constant  Value=150000
  Constant1 : Constant  Value=8000
  Product : Product
  Product1 : Product
  Sum : Sum  Inputs=--
  Mating Torque : Outport
  wires:
  Omega/1 -> Product1/1
  EA/1 -> Product/2
  Sum/1 -> Mating Torque/1
  Product1/1 -> Sum/2
  Product/1 -> Sum/1
  Constant1/1 -> Product1/2
  Constant/1 -> Product/1

== system Robot4_SDT/Tiles/Tile1/Variant Subsystem/Starting Position/massless connection body ==
  in1 : Inport  PortDimensions=18
  in2 : Inport  Port=2  PortDimensions=6
  Demux : Demux  Outputs=[ 6 18]
  Gain : RCTblocks/Uncertain State Space  Tag=USS  USystem=uss(KIN)  UValue=[]  X0=[]  uX0=[]
  Mux : Mux  Inputs=[ 18 6]
  out1 : Outport
  out2 : Outport  Port=2
  wires:
  Mux/1 -> Gain/1
  Gain/1 -> Demux/1
  in1/1 -> Mux/1
  Demux/1 -> out1/1
  in2/1 -> Mux/2
  Demux/2 -> out2/1

== system Robot4_SDT/Tiles/Tile2/Variant Subsystem/Depose/Force ==
  pos : Inport
  vel : Inport  Port=2
  Constant : Constant  Value=K_tile_force
  Constant1 : Constant  Value=C_tile_force
  Product : Product
  Product1 : Product
  Sum : Sum  Inputs=--
  Mating : Outport
  wires:
  Constant/1 -> Product/1
  Constant1/1 -> Product1/2
  Product/1 -> Sum/1
  Product1/1 -> Sum/2
  Sum/1 -> Mating/1
  pos/1 -> Product/2
  vel/1 -> Product1/1

== system Robot4_SDT/Tiles/Tile2/Variant Subsystem/Depose/Torque ==
  EA : Inport
  Omega : Inport  Port=2
  Constant : Constant  Value=K_tile_torque
  Constant1 : Constant  Value=C_tile_torque
  Product : Product
  Product1 : Product
  Sum : Sum  Inputs=--
  Mating : Outport
  wires:
  Constant/1 -> Product/1
  Constant1/1 -> Product1/2
  Product/1 -> Sum/1
  Product1/1 -> Sum/2
  Sum/1 -> Mating/1
  EA/1 -> Product/2
  Omega/1 -> Product1/1

== system Robot4_SDT/Tiles/Tile2/Variant Subsystem/Depose/massless connection body ==
  in1 : Inport  PortDimensions=18
  in2 : Inport  Port=2  PortDimensions=6
  Demux : Demux  Outputs=[ 6 18]
  Gain : RCTblocks/Uncertain State Space  Tag=USS  USystem=uss(KIN)  UValue=[]  X0=[]  uX0=[]
  Mux : Mux  Inputs=[ 18 6]
  out1 : Outport
  out2 : Outport  Port=2
  wires:
  Mux/1 -> Gain/1
  Gain/1 -> Demux/1
  in1/1 -> Mux/1
  Demux/1 -> out1/1
  in2/1 -> Mux/2
  Demux/2 -> out2/1

== system Robot4_SDT/Tiles/Tile2/Variant Subsystem/Grab/Force ==
  pos : Inport
  vel : Inport  Port=2
  Constant : Constant  Value=K_tile_force
  Constant1 : Constant  Value=C_tile_force
  Product : Product
  Product1 : Product
  Sum : Sum  Inputs=--
  Mating : Outport
  wires:
  vel/1 -> Product1/1
  pos/1 -> Product/2
  Sum/1 -> Mating/1
  Product1/1 -> Sum/2
  Product/1 -> Sum/1
  Constant1/1 -> Product1/2
  Constant/1 -> Product/1

== system Robot4_SDT/Tiles/Tile2/Variant Subsystem/Grab/Torque ==
  EA : Inport
  Omega : Inport  Port=2
  Constant : Constant  Value=K_tile_torque
  Constant1 : Constant  Value=C_tile_torque
  Product : Product
  Product1 : Product
  Sum : Sum  Inputs=--
  Mating : Outport
  wires:
  Omega/1 -> Product1/1
  EA/1 -> Product/2
  Sum/1 -> Mating/1
  Product1/1 -> Sum/2
  Product/1 -> Sum/1
  Constant1/1 -> Product1/2
  Constant/1 -> Product/1

== system Robot4_SDT/Tiles/Tile2/Variant Subsystem/Grab/massless connection body ==
  in1 : Inport  PortDimensions=18
  in2 : Inport  Port=2  PortDimensions=6
  Demux : Demux  Outputs=[ 6 18]
  Gain : RCTblocks/Uncertain State Space  Tag=USS  USystem=uss(KIN)  UValue=[]  X0=[]  uX0=[]
  Mux : Mux  Inputs=[ 18 6]
  out1 : Outport
  out2 : Outport  Port=2
  wires:
  Demux/2 -> out2/1
  in2/1 -> Mux/2
  Demux/1 -> out1/1
  in1/1 -> Mux/1
  Gain/1 -> Demux/1
  Mux/1 -> Gain/1

== system Robot4_SDT/Tiles/Tile2/Variant Subsystem/Starting Position/Force ==
  pos : Inport
  vel : Inport  Port=2
  Constant : Constant  Value=150000
  Constant1 : Constant  Value=8000
  Product : Product
  Product1 : Product
  Sum : Sum  Inputs=--
  Mating Force : Outport
  wires:
  vel/1 -> Product1/1
  pos/1 -> Product/2
  Sum/1 -> Mating Force/1
  Product1/1 -> Sum/2
  Product/1 -> Sum/1
  Constant1/1 -> Product1/2
  Constant/1 -> Product/1

== system Robot4_SDT/Tiles/Tile2/Variant Subsystem/Starting Position/Torque ==
  EA : Inport
  Omega : Inport  Port=2
  Constant : Constant  Value=150000
  Constant1 : Constant  Value=8000
  Product : Product
  Product1 : Product
  Sum : Sum  Inputs=--
  Mating Torque : Outport
  wires:
  Constant/1 -> Product/1
  Constant1/1 -> Product1/2
  Product/1 -> Sum/1
  Product1/1 -> Sum/2
  Sum/1 -> Mating Torque/1
  EA/1 -> Product/2
  Omega/1 -> Product1/1

== system Robot4_SDT/Tiles/Tile2/Variant Subsystem/Starting Position/massless connection body ==
  in1 : Inport  PortDimensions=18
  in2 : Inport  Port=2  PortDimensions=6
  Demux : Demux  Outputs=[ 6 18]
  Gain : RCTblocks/Uncertain State Space  Tag=USS  USystem=uss(KIN)  UValue=[]  X0=[]  uX0=[]
  Mux : Mux  Inputs=[ 18 6]
  out1 : Outport
  out2 : Outport  Port=2
  wires:
  Demux/2 -> out2/1
  in2/1 -> Mux/2
  Demux/1 -> out1/1
  in1/1 -> Mux/1
  Gain/1 -> Demux/1
  Mux/1 -> Gain/1

== system Robot4_SDT/Tiles/Tile3/Variant Subsystem/Depose/Force ==
  pos : Inport
  vel : Inport  Port=2
  Constant : Constant  Value=K_tile_force
  Constant1 : Constant  Value=C_tile_force
  Product : Product
  Product1 : Product
  Sum : Sum  Inputs=--
  Mating : Outport
  wires:
  vel/1 -> Product1/1
  pos/1 -> Product/2
  Sum/1 -> Mating/1
  Product1/1 -> Sum/2
  Product/1 -> Sum/1
  Constant1/1 -> Product1/2
  Constant/1 -> Product/1

== system Robot4_SDT/Tiles/Tile3/Variant Subsystem/Depose/Torque ==
  EA : Inport
  Omega : Inport  Port=2
  Constant : Constant  Value=K_tile_torque
  Constant1 : Constant  Value=C_tile_torque
  Product : Product
  Product1 : Product
  Sum : Sum  Inputs=--
  Mating : Outport
  wires:
  Omega/1 -> Product1/1
  EA/1 -> Product/2
  Sum/1 -> Mating/1
  Product1/1 -> Sum/2
  Product/1 -> Sum/1
  Constant1/1 -> Product1/2
  Constant/1 -> Product/1

== system Robot4_SDT/Tiles/Tile3/Variant Subsystem/Depose/massless connection body ==
  in1 : Inport  PortDimensions=18
  in2 : Inport  Port=2  PortDimensions=6
  Demux : Demux  Outputs=[ 6 18]
  Gain : RCTblocks/Uncertain State Space  Tag=USS  USystem=uss(KIN)  UValue=[]  X0=[]  uX0=[]
  Mux : Mux  Inputs=[ 18 6]
  out1 : Outport
  out2 : Outport  Port=2
  wires:
  Demux/2 -> out2/1
  in2/1 -> Mux/2
  Demux/1 -> out1/1
  in1/1 -> Mux/1
  Gain/1 -> Demux/1
  Mux/1 -> Gain/1

== system Robot4_SDT/Tiles/Tile3/Variant Subsystem/Grab/Force ==
  pos : Inport
  vel : Inport  Port=2
  Constant : Constant  Value=K_tile_force
  Constant1 : Constant  Value=C_tile_force
  Product : Product
  Product1 : Product
  Sum : Sum  Inputs=--
  Mating : Outport
  wires:
  Constant/1 -> Product/1
  Constant1/1 -> Product1/2
  Product/1 -> Sum/1
  Product1/1 -> Sum/2
  Sum/1 -> Mating/1
  pos/1 -> Product/2
  vel/1 -> Product1/1

== system Robot4_SDT/Tiles/Tile3/Variant Subsystem/Grab/Torque ==
  EA : Inport
  Omega : Inport  Port=2
  Constant : Constant  Value=K_tile_torque
  Constant1 : Constant  Value=C_tile_torque
  Product : Product
  Product1 : Product
  Sum : Sum  Inputs=--
  Mating : Outport
  wires:
  Constant/1 -> Product/1
  Constant1/1 -> Product1/2
  Product/1 -> Sum/1
  Product1/1 -> Sum/2
  Sum/1 -> Mating/1
  EA/1 -> Product/2
  Omega/1 -> Product1/1

== system Robot4_SDT/Tiles/Tile3/Variant Subsystem/Grab/massless connection body ==
  in1 : Inport  PortDimensions=18
  in2 : Inport  Port=2  PortDimensions=6
  Demux : Demux  Outputs=[ 6 18]
  Gain : RCTblocks/Uncertain State Space  Tag=USS  USystem=uss(KIN)  UValue=[]  X0=[]  uX0=[]
  Mux : Mux  Inputs=[ 18 6]
  out1 : Outport
  out2 : Outport  Port=2
  wires:
  Mux/1 -> Gain/1
  Gain/1 -> Demux/1
  in1/1 -> Mux/1
  Demux/1 -> out1/1
  in2/1 -> Mux/2
  Demux/2 -> out2/1

== system Robot4_SDT/Tiles/Tile3/Variant Subsystem/Starting Position/Force ==
  pos : Inport
  vel : Inport  Port=2
  Constant : Constant  Value=150000
  Constant1 : Constant  Value=8000
  Product : Product
  Product1 : Product
  Sum : Sum  Inputs=--
  Mating Force : Outport
  wires:
  Constant/1 -> Product/1
  Constant1/1 -> Product1/2
  Product/1 -> Sum/1
  Product1/1 -> Sum/2
  Sum/1 -> Mating Force/1
  pos/1 -> Product/2
  vel/1 -> Product1/1

== system Robot4_SDT/Tiles/Tile3/Variant Subsystem/Starting Position/Torque ==
  EA : Inport
  Omega : Inport  Port=2
  Constant : Constant  Value=150000
  Constant1 : Constant  Value=8000
  Product : Product
  Product1 : Product
  Sum : Sum  Inputs=--
  Mating Torque : Outport
  wires:
  Omega/1 -> Product1/1
  EA/1 -> Product/2
  Sum/1 -> Mating Torque/1
  Product1/1 -> Sum/2
  Product/1 -> Sum/1
  Constant1/1 -> Product1/2
  Constant/1 -> Product/1

== system Robot4_SDT/Tiles/Tile3/Variant Subsystem/Starting Position/massless connection body ==
  in1 : Inport  PortDimensions=18
  in2 : Inport  Port=2  PortDimensions=6
  Demux : Demux  Outputs=[ 6 18]
  Gain : RCTblocks/Uncertain State Space  Tag=USS  USystem=uss(KIN)  UValue=[]  X0=[]  uX0=[]
  Mux : Mux  Inputs=[ 18 6]
  out1 : Outport
  out2 : Outport  Port=2
  wires:
  Mux/1 -> Gain/1
  Gain/1 -> Demux/1
  in1/1 -> Mux/1
  Demux/1 -> out1/1
  in2/1 -> Mux/2
  Demux/2 -> out2/1

== system Robot4_SDT/Tiles/Tile4/Variant Subsystem/Depose/Force ==
  pos : Inport
  vel : Inport  Port=2
  Constant : Constant  Value=K_tile_force
  Constant1 : Constant  Value=C_tile_force
  Product : Product
  Product1 : Product
  Sum : Sum  Inputs=--
  Mating : Outport
  wires:
  Constant/1 -> Product/1
  Constant1/1 -> Product1/2
  Product/1 -> Sum/1
  Product1/1 -> Sum/2
  Sum/1 -> Mating/1
  pos/1 -> Product/2
  vel/1 -> Product1/1

== system Robot4_SDT/Tiles/Tile4/Variant Subsystem/Depose/Torque ==
  EA : Inport
  Omega : Inport  Port=2
  Constant : Constant  Value=K_tile_torque
  Constant1 : Constant  Value=C_tile_torque
  Product : Product
  Product1 : Product
  Sum : Sum  Inputs=--
  Mating : Outport
  wires:
  Constant/1 -> Product/1
  Constant1/1 -> Product1/2
  Product/1 -> Sum/1
  Product1/1 -> Sum/2
  Sum/1 -> Mating/1
  EA/1 -> Product/2
  Omega/1 -> Product1/1

== system Robot4_SDT/Tiles/Tile4/Variant Subsystem/Depose/massless connection body ==
  in1 : Inport  PortDimensions=18
  in2 : Inport  Port=2  PortDimensions=6
  Demux : Demux  Outputs=[ 6 18]
  Gain : RCTblocks/Uncertain State Space  Tag=USS  USystem=uss(KIN)  UValue=[]  X0=[]  uX0=[]
  Mux : Mux  Inputs=[ 18 6]
  out1 : Outport
  out2 : Outport  Port=2
  wires:
  Mux/1 -> Gain/1
  Gain/1 -> Demux/1
  in1/1 -> Mux/1
  Demux/1 -> out1/1
  in2/1 -> Mux/2
  Demux/2 -> out2/1

== system Robot4_SDT/Tiles/Tile4/Variant Subsystem/Grab/Force ==
  pos : Inport
  vel : Inport  Port=2
  Constant : Constant  Value=K_tile_force
  Constant1 : Constant  Value=C_tile_force
  Product : Product
  Product1 : Product
  Sum : Sum  Inputs=--
  Mating : Outport
  wires:
  vel/1 -> Product1/1
  pos/1 -> Product/2
  Sum/1 -> Mating/1
  Product1/1 -> Sum/2
  Product/1 -> Sum/1
  Constant1/1 -> Product1/2
  Constant/1 -> Product/1

== system Robot4_SDT/Tiles/Tile4/Variant Subsystem/Grab/Torque ==
  EA : Inport
  Omega : Inport  Port=2
  Constant : Constant  Value=K_tile_torque
  Constant1 : Constant  Value=C_tile_torque
  Product : Product
  Product1 : Product
  Sum : Sum  Inputs=--
  Mating : Outport
  wires:
  Omega/1 -> Product1/1
  EA/1 -> Product/2
  Sum/1 -> Mating/1
  Product1/1 -> Sum/2
  Product/1 -> Sum/1
  Constant1/1 -> Product1/2
  Constant/1 -> Product/1

== system Robot4_SDT/Tiles/Tile4/Variant Subsystem/Grab/massless connection body ==
  in1 : Inport  PortDimensions=18
  in2 : Inport  Port=2  PortDimensions=6
  Demux : Demux  Outputs=[ 6 18]
  Gain : RCTblocks/Uncertain State Space  Tag=USS  USystem=uss(KIN)  UValue=[]  X0=[]  uX0=[]
  Mux : Mux  Inputs=[ 18 6]
  out1 : Outport
  out2 : Outport  Port=2
  wires:
  Demux/2 -> out2/1
  in2/1 -> Mux/2
  Demux/1 -> out1/1
  in1/1 -> Mux/1
  Gain/1 -> Demux/1
  Mux/1 -> Gain/1

== system Robot4_SDT/Tiles/Tile4/Variant Subsystem/Starting Position/Force ==
  pos : Inport
  vel : Inport  Port=2
  Constant : Constant  Value=150000
  Constant1 : Constant  Value=8000
  Product : Product
  Product1 : Product
  Sum : Sum  Inputs=--
  Mating Force : Outport
  wires:
  vel/1 -> Product1/1
  pos/1 -> Product/2
  Sum/1 -> Mating Force/1
  Product1/1 -> Sum/2
  Product/1 -> Sum/1
  Constant1/1 -> Product1/2
  Constant/1 -> Product/1

== system Robot4_SDT/Tiles/Tile4/Variant Subsystem/Starting Position/Torque ==
  EA : Inport
  Omega : Inport  Port=2
  Constant : Constant  Value=150000
  Constant1 : Constant  Value=8000
  Product : Product
  Product1 : Product
  Sum : Sum  Inputs=--
  Mating Torque : Outport
  wires:
  Constant/1 -> Product/1
  Constant1/1 -> Product1/2
  Product/1 -> Sum/1
  Product1/1 -> Sum/2
  Sum/1 -> Mating Torque/1
  EA/1 -> Product/2
  Omega/1 -> Product1/1

== system Robot4_SDT/Tiles/Tile4/Variant Subsystem/Starting Position/massless connection body ==
  in1 : Inport  PortDimensions=18
  in2 : Inport  Port=2  PortDimensions=6
  Demux : Demux  Outputs=[ 6 18]
  Gain : RCTblocks/Uncertain State Space  Tag=USS  USystem=uss(KIN)  UValue=[]  X0=[]  uX0=[]
  Mux : Mux  Inputs=[ 18 6]
  out1 : Outport
  out2 : Outport  Port=2
  wires:
  Demux/2 -> out2/1
  in2/1 -> Mux/2
  Demux/1 -> out1/1
  in1/1 -> Mux/1
  Gain/1 -> Demux/1
  Mux/1 -> Gain/1

== system Robot4_SDT/Tiles/Tile5/Variant Subsystem/Depose/Force ==
  pos : Inport
  vel : Inport  Port=2
  Constant : Constant  Value=K_tile_force
  Constant1 : Constant  Value=C_tile_force
  Product : Product
  Product1 : Product
  Sum : Sum  Inputs=--
  Mating : Outport
  wires:
  vel/1 -> Product1/1
  pos/1 -> Product/2
  Sum/1 -> Mating/1
  Product1/1 -> Sum/2
  Product/1 -> Sum/1
  Constant1/1 -> Product1/2
  Constant/1 -> Product/1

== system Robot4_SDT/Tiles/Tile5/Variant Subsystem/Depose/Torque ==
  EA : Inport
  Omega : Inport  Port=2
  Constant : Constant  Value=K_tile_torque
  Constant1 : Constant  Value=C_tile_torque
  Product : Product
  Product1 : Product
  Sum : Sum  Inputs=--
  Mating : Outport
  wires:
  Omega/1 -> Product1/1
  EA/1 -> Product/2
  Sum/1 -> Mating/1
  Product1/1 -> Sum/2
  Product/1 -> Sum/1
  Constant1/1 -> Product1/2
  Constant/1 -> Product/1

== system Robot4_SDT/Tiles/Tile5/Variant Subsystem/Depose/massless connection body ==
  in1 : Inport  PortDimensions=18
  in2 : Inport  Port=2  PortDimensions=6
  Demux : Demux  Outputs=[ 6 18]
  Gain : RCTblocks/Uncertain State Space  Tag=USS  USystem=uss(KIN)  UValue=[]  X0=[]  uX0=[]
  Mux : Mux  Inputs=[ 18 6]
  out1 : Outport
  out2 : Outport  Port=2
  wires:
  Demux/2 -> out2/1
  in2/1 -> Mux/2
  Demux/1 -> out1/1
  in1/1 -> Mux/1
  Gain/1 -> Demux/1
  Mux/1 -> Gain/1

== system Robot4_SDT/Tiles/Tile5/Variant Subsystem/Grab/Force ==
  pos : Inport
  vel : Inport  Port=2
  Constant : Constant  Value=K_tile_force
  Constant1 : Constant  Value=C_tile_force
  Product : Product
  Product1 : Product
  Sum : Sum  Inputs=--
  Mating : Outport
  wires:
  Constant/1 -> Product/1
  Constant1/1 -> Product1/2
  Product/1 -> Sum/1
  Product1/1 -> Sum/2
  Sum/1 -> Mating/1
  pos/1 -> Product/2
  vel/1 -> Product1/1

== system Robot4_SDT/Tiles/Tile5/Variant Subsystem/Grab/Torque ==
  EA : Inport
  Omega : Inport  Port=2
  Constant : Constant  Value=K_tile_torque
  Constant1 : Constant  Value=C_tile_torque
  Product : Product
  Product1 : Product
  Sum : Sum  Inputs=--
  Mating : Outport
  wires:
  Constant/1 -> Product/1
  Constant1/1 -> Product1/2
  Product/1 -> Sum/1
  Product1/1 -> Sum/2
  Sum/1 -> Mating/1
  EA/1 -> Product/2
  Omega/1 -> Product1/1

== system Robot4_SDT/Tiles/Tile5/Variant Subsystem/Grab/massless connection body ==
  in1 : Inport  PortDimensions=18
  in2 : Inport  Port=2  PortDimensions=6
  Demux : Demux  Outputs=[ 6 18]
  Gain : RCTblocks/Uncertain State Space  Tag=USS  USystem=uss(KIN)  UValue=[]  X0=[]  uX0=[]
  Mux : Mux  Inputs=[ 18 6]
  out1 : Outport
  out2 : Outport  Port=2
  wires:
  Mux/1 -> Gain/1
  Gain/1 -> Demux/1
  in1/1 -> Mux/1
  Demux/1 -> out1/1
  in2/1 -> Mux/2
  Demux/2 -> out2/1

== system Robot4_SDT/Tiles/Tile5/Variant Subsystem/Starting Position/Force ==
  pos : Inport
  vel : Inport  Port=2
  Constant : Constant  Value=150000
  Constant1 : Constant  Value=8000
  Product : Product
  Product1 : Product
  Sum : Sum  Inputs=--
  Mating Force : Outport
  wires:
  Constant/1 -> Product/1
  Constant1/1 -> Product1/2
  Product/1 -> Sum/1
  Product1/1 -> Sum/2
  Sum/1 -> Mating Force/1
  pos/1 -> Product/2
  vel/1 -> Product1/1

== system Robot4_SDT/Tiles/Tile5/Variant Subsystem/Starting Position/Torque ==
  EA : Inport
  Omega : Inport  Port=2
  Constant : Constant  Value=150000
  Constant1 : Constant  Value=8000
  Product : Product
  Product1 : Product
  Sum : Sum  Inputs=--
  Mating Torque : Outport
  wires:
  Omega/1 -> Product1/1
  EA/1 -> Product/2
  Sum/1 -> Mating Torque/1
  Product1/1 -> Sum/2
  Product/1 -> Sum/1
  Constant1/1 -> Product1/2
  Constant/1 -> Product/1

== system Robot4_SDT/Tiles/Tile5/Variant Subsystem/Starting Position/massless connection body ==
  in1 : Inport  PortDimensions=18
  in2 : Inport  Port=2  PortDimensions=6
  Demux : Demux  Outputs=[ 6 18]
  Gain : RCTblocks/Uncertain State Space  Tag=USS  USystem=uss(KIN)  UValue=[]  X0=[]  uX0=[]
  Mux : Mux  Inputs=[ 18 6]
  out1 : Outport
  out2 : Outport  Port=2
  wires:
  Mux/1 -> Gain/1
  Gain/1 -> Demux/1
  in1/1 -> Mux/1
  Demux/1 -> out1/1
  in2/1 -> Mux/2
  Demux/2 -> out2/1

== system Robot4_SDT/Tiles/Tile6/Variant Subsystem/Depose/Force ==
  pos : Inport
  vel : Inport  Port=2
  Constant : Constant  Value=K_tile_force
  Constant1 : Constant  Value=C_tile_force
  Product : Product
  Product1 : Product
  Sum : Sum  Inputs=--
  Mating : Outport
  wires:
  Constant/1 -> Product/1
  Constant1/1 -> Product1/2
  Product/1 -> Sum/1
  Product1/1 -> Sum/2
  Sum/1 -> Mating/1
  pos/1 -> Product/2
  vel/1 -> Product1/1

== system Robot4_SDT/Tiles/Tile6/Variant Subsystem/Depose/Torque ==
  EA : Inport
  Omega : Inport  Port=2
  Constant : Constant  Value=K_tile_torque
  Constant1 : Constant  Value=C_tile_torque
  Product : Product
  Product1 : Product
  Sum : Sum  Inputs=--
  Mating : Outport
  wires:
  Constant/1 -> Product/1
  Constant1/1 -> Product1/2
  Product/1 -> Sum/1
  Product1/1 -> Sum/2
  Sum/1 -> Mating/1
  EA/1 -> Product/2
  Omega/1 -> Product1/1

== system Robot4_SDT/Tiles/Tile6/Variant Subsystem/Depose/massless connection body ==
  in1 : Inport  PortDimensions=18
  in2 : Inport  Port=2  PortDimensions=6
  Demux : Demux  Outputs=[ 6 18]
  Gain : RCTblocks/Uncertain State Space  Tag=USS  USystem=uss(KIN)  UValue=[]  X0=[]  uX0=[]
  Mux : Mux  Inputs=[ 18 6]
  out1 : Outport
  out2 : Outport  Port=2
  wires:
  Mux/1 -> Gain/1
  Gain/1 -> Demux/1
  in1/1 -> Mux/1
  Demux/1 -> out1/1
  in2/1 -> Mux/2
  Demux/2 -> out2/1

== system Robot4_SDT/Tiles/Tile6/Variant Subsystem/Grab/Force ==
  pos : Inport
  vel : Inport  Port=2
  Constant : Constant  Value=K_tile_force
  Constant1 : Constant  Value=C_tile_force
  Product : Product
  Product1 : Product
  Sum : Sum  Inputs=--
  Mating : Outport
  wires:
  vel/1 -> Product1/1
  pos/1 -> Product/2
  Sum/1 -> Mating/1
  Product1/1 -> Sum/2
  Product/1 -> Sum/1
  Constant1/1 -> Product1/2
  Constant/1 -> Product/1

== system Robot4_SDT/Tiles/Tile6/Variant Subsystem/Grab/Torque ==
  EA : Inport
  Omega : Inport  Port=2
  Constant : Constant  Value=K_tile_torque
  Constant1 : Constant  Value=C_tile_torque
  Product : Product
  Product1 : Product
  Sum : Sum  Inputs=--
  Mating : Outport
  wires:
  Omega/1 -> Product1/1
  EA/1 -> Product/2
  Sum/1 -> Mating/1
  Product1/1 -> Sum/2
  Product/1 -> Sum/1
  Constant1/1 -> Product1/2
  Constant/1 -> Product/1
